simulink model "VCU_ASW"  (R2018b)
settings: Solver=FixedStepAuto  StartTime=0.0  StopTime=10.0  RelTol=1e-3
settings Model: Creator=91698  LastModifiedBy=91698
settings SolverCC: AutoInsertRateTranBlk=on
settings OptimizationCC: DefaultParameterBehavior=Inlined  EnhancedBackFolding=on  PassReuseOutputArgsAs=Individual arguments  OptimizeBlockOrder=speed  DifferentSizesBufferReuse=on  OptimizationCustomize=off
settings DebuggingCC: ParameterTunabilityLossMsg=error
settings HardwareCC: ProdBitPerPointer=32  ProdBitPerSizeT=32  ProdBitPerPtrDiffT=32  ProdLargestAtomicInteger=Long  ProdLargestAtomicFloat=Double  ProdEndianess=BigEndian  ProdWordSize=32  ProdHWDeviceType=Freescale->32-bit PowerPC
settings SFSimCC: MATLABDynamicMemAlloc=off
settings RTWCC: SystemTargetFile=ert.tlc  GenCodeOnly=on  TemplateMakefile=ert_default_tmf  GenerateReport=on  IncludeHyperlinkInReport=on  LaunchReport=on  GenerateTraceInfo=on  GenerateTraceReport=on  GenerateTraceReportSl=on  GenerateTraceReportSf=on  GenerateTraceReportEml=on
settings CodeAppCC: ForceParamTrailComments=on  IgnoreCustomStorageClasses=off  OperatorAnnotations=on  SimulinkDataObjDesc=on  SFDataObjDesc=on  InsertBlockDesc=on
settings ERTTargetCC: TargetLangStandard=C99 (ISO)  GenerateSampleERTMain=on  InlinedParameterPlacement=NonHierarchical  ERTCustomFileTemplate=example_file_process.tlc

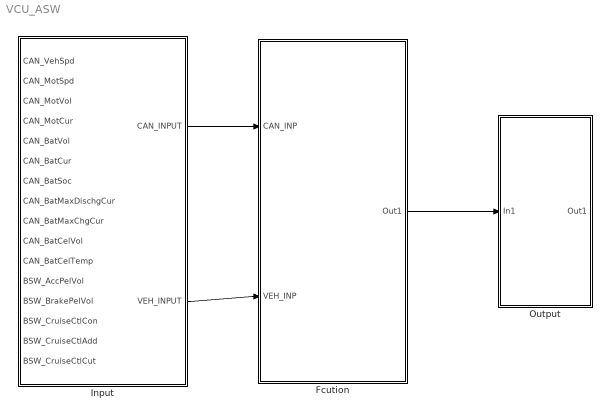
== system VCU_ASW ==
  Fcution : Subsystem
  Input : Subsystem
  Output : Subsystem
  wires:
  Input/2(VEH_INPUT) -> Fcution/2(VEH_INP)
  Input/1(CAN_INPUT) -> Fcution/1(CAN_INP)
  Fcution/1(Out1) -> Output/1(In1)

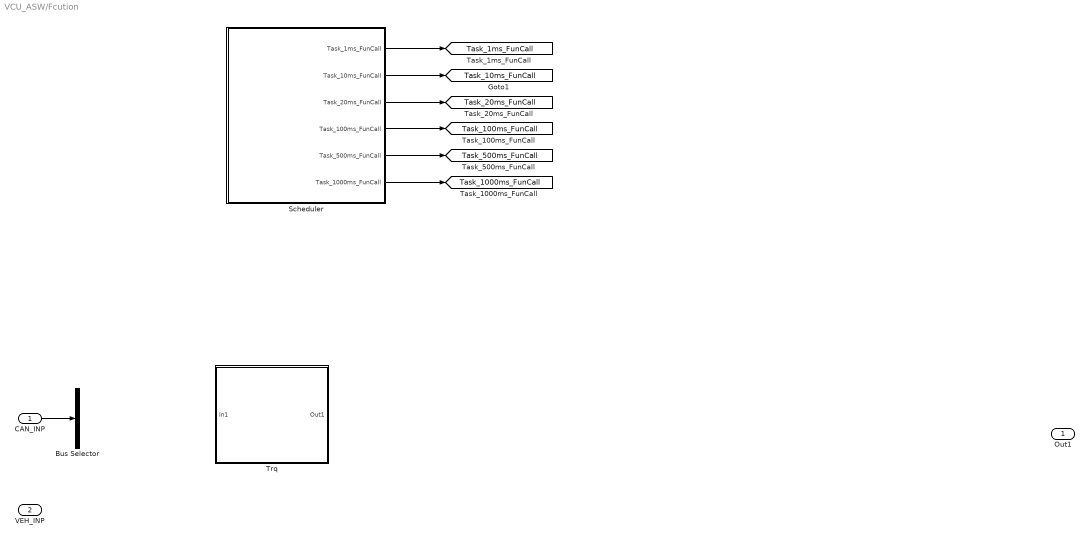
== system VCU_ASW/Fcution ==
  CAN_INP : Inport
  VEH_INP : Inport  Port=2
  Bus Selector : BusSelector  OutputSignals=signal1,signal2
  Scheduler : Subsystem
  Trq : Subsystem  TreatAsAtomicUnit=on
  Out1 : Outport
  tag scope: Task_1000ms_FunCall=global, Task_100ms_FunCall=global, Task_10ms_FunCall=global, Task_1ms_FunCall=global, Task_20ms_FunCall=global, Task_500ms_FunCall=global
  wires:
  Scheduler/1(Task_1ms_FunCall) -> [Task_1ms_FunCall]
  Scheduler/2(Task_10ms_FunCall) -> [Task_10ms_FunCall]
  Scheduler/3(Task_20ms_FunCall) -> [Task_20ms_FunCall]
  Scheduler/4(Task_100ms_FunCall) -> [Task_100ms_FunCall]
  Scheduler/5(Task_500ms_FunCall) -> [Task_500ms_FunCall]
  Scheduler/6(Task_1000ms_FunCall) -> [Task_1000ms_FunCall]
  CAN_INP/1 -> Bus Selector/1

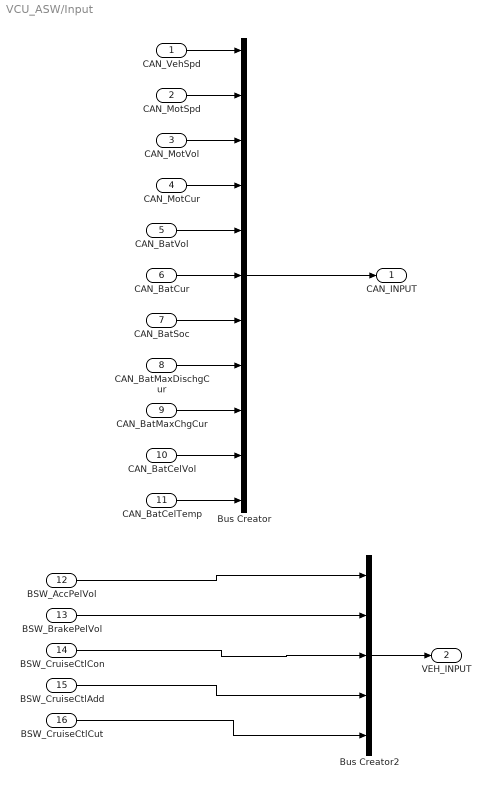
== system VCU_ASW/Input ==
  CAN_VehSpd : Inport
  CAN_MotSpd : Inport  Port=2
  CAN_MotVol : Inport  Port=3
  CAN_MotCur : Inport  Port=4
  CAN_BatVol : Inport  Port=5
  CAN_BatCur : Inport  Port=6
  CAN_BatSoc : Inport  Port=7
  CAN_BatMaxDischgCur : Inport  Port=8
  CAN_BatMaxChgCur : Inport  Port=9
  CAN_BatCelVol : Inport  Port=10
  CAN_BatCelTemp : Inport  Port=11
  BSW_AccPelVol : Inport  Port=12
  BSW_BrakePelVol : Inport  Port=13
  BSW_CruiseCtlCon : Inport  Port=14
  BSW_CruiseCtlAdd : Inport  Port=15
  BSW_CruiseCtlCut : Inport  Port=16
  Bus Creator : BusCreator  Inputs=11
  Bus Creator2 : BusCreator  Inputs=5
  CAN_INPUT : Outport
  VEH_INPUT : Outport  Port=2
  wires:
  CAN_VehSpd/1 -> Bus Creator/1
  CAN_MotSpd/1 -> Bus Creator/2
  CAN_MotVol/1 -> Bus Creator/3
  CAN_MotCur/1 -> Bus Creator/4
  CAN_BatVol/1 -> Bus Creator/5
  CAN_BatCur/1 -> Bus Creator/6
  CAN_BatSoc/1 -> Bus Creator/7
  CAN_BatMaxDischgCur/1 -> Bus Creator/8
  CAN_BatMaxChgCur/1 -> Bus Creator/9
  CAN_BatCelVol/1 -> Bus Creator/10
  CAN_BatCelTemp/1 -> Bus Creator/11
  Bus Creator/1 -> CAN_INPUT/1
  BSW_AccPelVol/1 -> Bus Creator2/1
  BSW_BrakePelVol/1 -> Bus Creator2/2
  BSW_CruiseCtlCon/1 -> Bus Creator2/3
  BSW_CruiseCtlAdd/1 -> Bus Creator2/4
  BSW_CruiseCtlCut/1 -> Bus Creator2/5
  Bus Creator2/1 -> VEH_INPUT/1

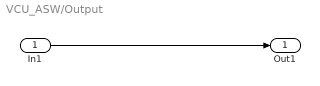
== system VCU_ASW/Output ==
  In1 : Inport
  Out1 : Outport
  wires:
  In1/1 -> Out1/1

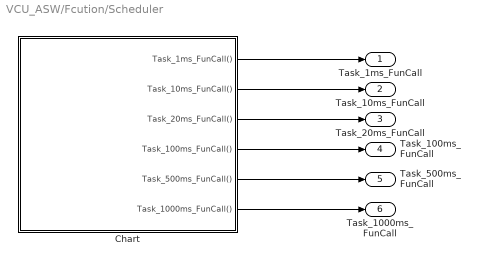
== system VCU_ASW/Fcution/Scheduler ==
  Chart : Stateflow chart  TreatAsAtomicUnit=on
  Task_1ms_FunCall : Outport
  Task_10ms_FunCall : Outport  Port=2
  Task_20ms_FunCall : Outport  Port=3
  Task_100ms_FunCall : Outport  Port=4
  Task_500ms_FunCall : Outport  Port=5
  Task_1000ms_FunCall : Outport  Port=6
  wires:
  Chart/1(Task_1ms_FunCall()) -> Task_1ms_FunCall/1
  Chart/2(Task_10ms_FunCall()) -> Task_10ms_FunCall/1
  Chart/3(Task_20ms_FunCall()) -> Task_20ms_FunCall/1
  Chart/4(Task_100ms_FunCall()) -> Task_100ms_FunCall/1
  Chart/5(Task_500ms_FunCall()) -> Task_500ms_FunCall/1
  Chart/6(Task_1000ms_FunCall()) -> Task_1000ms_FunCall/1

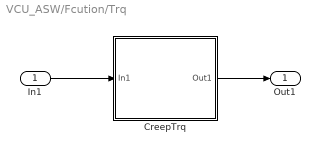
== system VCU_ASW/Fcution/Trq ==
  In1 : Inport
  CreepTrq : Subsystem
  Out1 : Outport
  wires:
  In1/1 -> CreepTrq/1(In1)
  CreepTrq/1(Out1) -> Out1/1

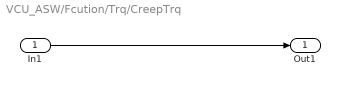
== system VCU_ASW/Fcution/Trq/CreepTrq ==
  In1 : Inport
  Out1 : Outport
  wires:
  In1/1 -> Out1/1

== stateflow chart VCU_ASW/Fcution/Scheduler/Chart ==
  (default) -> (junction 1) : {Task_1ms_FunCall;}
  (junction 1) -> (junction 9) : {TimeCnt++;}
  (junction 9) -> (junction 14) [order 1] : [TimeCnt%%10==0]
  (junction 9) -> (junction 17) [order 2]
  (junction 14) -> (junction 18) : {Task_10ms_FunCall;}
  (junction 18) -> (junction 17)
  (junction 17) -> (junction 22)
  (junction 22) -> (junction 23) [order 1] : [TimeCnt%%20==0]
  (junction 22) -> (junction 28) [order 2]
  (junction 23) -> (junction 26) : {Task_20ms_FunCall;}
  (junction 26) -> (junction 28)
  (junction 28) -> (junction 35)
  (junction 35) -> (junction 34) [order 1] : [TimeCnt%%100==0]
  (junction 35) -> (junction 33) [order 2]
  (junction 34) -> (junction 31) : {Task_100ms_FunCall;}
  (junction 31) -> (junction 33)
  (junction 33) -> (junction 44)
  (junction 44) -> (junction 43) [order 1] : [TimeCnt%%500==0]
  (junction 44) -> (junction 42) [order 2]
  (junction 43) -> (junction 40) : {Task_500ms_FunCall;}
  (junction 40) -> (junction 42)
  (junction 42) -> (junction 53)
  (junction 53) -> (junction 52) [order 1] : [TimeCnt%%1000==0]
  (junction 53) -> (junction 51) [order 2]
  (junction 52) -> (junction 49) : {Task_1000ms_FunCall;}
  (junction 49) -> (junction 51)
  (junction 51) -> (junction 58)
  data: TimeCnt local uint32
  events: Task_1ms_FunCall output FUNCTION_CALL_EVENT; Task_10ms_FunCall output FUNCTION_CALL_EVENT; Task_20ms_FunCall output FUNCTION_CALL_EVENT; Task_100ms_FunCall output FUNCTION_CALL_EVENT; Task_500ms_FunCall output FUNCTION_CALL_EVENT; Task_1000ms_FunCall output FUNCTION_CALL_EVENT
